simulink model "fxpdemo_diff"  (Simulink 5.0)
settings: Solver=ode5  SolverMode=SingleTasking  StartTime=0.0  StopTime=10  FixedStep=SampleTime/5  RelTol=1e-3  AbsTol=1e-6
PreLoadFcn:
  | preload_diff
values from neighbouring files (symbols this model uses):
  PoleZ = 0.85    [preload_diff.m]    (also in preload_lead_lag.m = exp( SampleTime * PoleS     ))
  SampleTime = 0.05    [preload_diff.m]    (also in preload_integrate.m; preload_lead_lag.m; preload_state_space.m = 0.01)
libraries: fixpt_lib_4 x7, simulink x1, fixpt_lib_3p1 x1
settings Model: RequirementInfo=9  CovMetricSettings=d  MinMaxOverflowLogging=MinMaxAndOverflow  Creator=andyb  LastModifiedBy=andyb  ExtModeTrigMode=oneshot  ExtModeArmWhenConnect=off  ExtModeAutoUpdateStatusClock=off  LimitDataPoints=off  IntegerOverflowMsg=none  ParameterDowncastMsg=warning  ParameterOverflowMsg=warning  ParameterPrecisionLossMsg=none  BooleanDataType=off  RTWOptions="-aEnforceIntegerDowncast=1 -aExtMode=0 -aExtModeTesting=0 -aFoldNonRolledExpr=1 -aForceParamTrailComments=0 -aGenRTModel=1 -aGenerateComments=1 -aGenerateReport=0 -aIgnoreCustomStorageClasses=1 -aIncHierarchyInIds=0 -aInlineInvariantSignals=0 -aLocalBlockOutputs=1 -aLogVarNameModifier=\"rt_\" -aRTWVerbose=1 -aRollThreshold=5 -aShowEliminatedStatements=1"

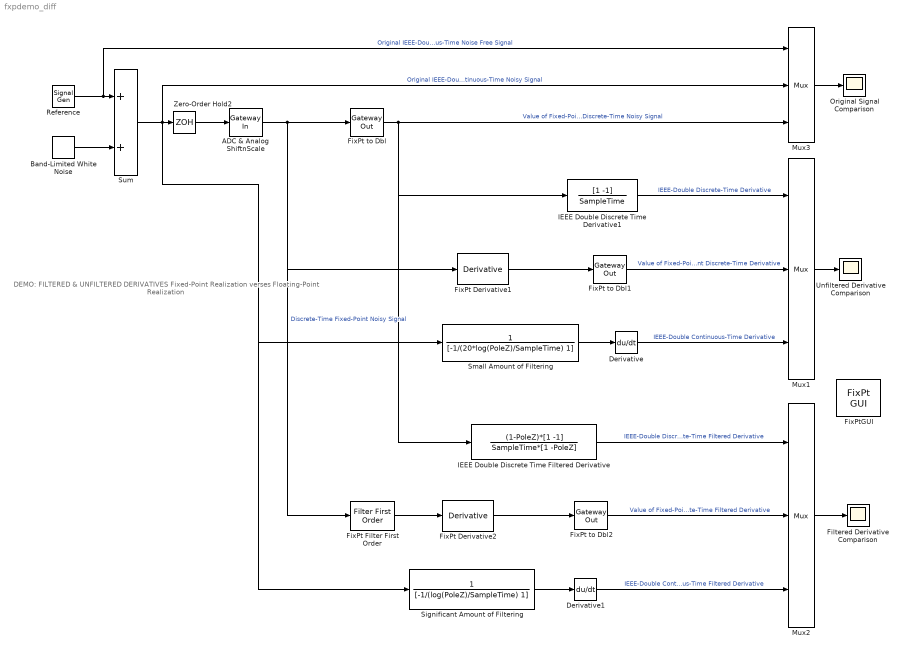
== system fxpdemo_diff ==
  note: DEMO:
      |
      | FILTERED &
      | UNFILTERED
      | DERIVATIVES
      |
      | Fixed-Point Realization
      | verses
      | Floating-Point Realization
  ADC & Analog ShiftnScale : fixpt_lib_4/Data Type/Gateway In  InRealWorld=Real World Value  OutputDataTypeScalingMode=Specify via dialog  OutDataType=sfix(16)  OutScaling=2^-9  RndMeth=Nearest  DoSatur=on
      settings: LockScale=on
  Band-Limited White Noise : simulink/Sources/Band-Limited White Noise  Cov=[0.0000005]  Ts=SampleTime/5  seed=[23341]
  Derivative : Derivative
  Derivative1 : Derivative
  Filtered Derivative Comparison : Scope
      settings: TickLabels=on  YMin=-3  YMax=3  SaveName=FiltDerivCompare
  FixPt Derivative1 : fixpt_lib_4/Calculus/Derivative  gainval=1.0  ICPrevScaledInput=0.0  OutDataType=sfix(16)  OutScaling=2^-10  DoSatur=off
  FixPt Derivative2 : fixpt_lib_4/Calculus/Derivative  gainval=1.0  ICPrevScaledInput=0.0  OutDataType=sfix(16)  OutScaling=2^-10  DoSatur=off
  FixPt Filter First Order : fixpt_lib_4/Filters/Filter First Order  PoleZ=PoleZ  ICPrevOutput=0.0  DoSatur=off
  FixPt to Dbl : fixpt_lib_4/Data Type/Gateway Out  OutRealWorld=Real World Value  OutBuiltInType=double  DoSatur=off
  FixPt to Dbl1 : fixpt_lib_4/Data Type/Gateway Out  OutRealWorld=Real World Value  OutBuiltInType=double  DoSatur=off
  FixPt to Dbl2 : fixpt_lib_4/Data Type/Gateway Out  OutRealWorld=Real World Value  OutBuiltInType=double  DoSatur=off
  FixPtGUI : fixpt_lib_3p1/FixPt GUI
  IEEE Double Discrete Time Derivative1 : DiscreteFilter  Numerator=[1 -1]  Denominator=SampleTime  SampleTime=SampleTime
  IEEE Double Discrete Time Filtered Derivative : DiscreteFilter  Numerator=(1-PoleZ)*[1 -1]  Denominator=SampleTime*[1 -PoleZ]  SampleTime=SampleTime
  Mux1 : Mux  Inputs=3
  Mux2 : Mux  Inputs=3
  Mux3 : Mux  Inputs=3
  Original Signal Comparison : Scope
      settings: TickLabels=on  YMin=-4  YMax=4  SaveName=OrigSignalCompare
  Reference : SignalGenerator  Amplitude=3  Frequency=0.1*1
  Significant Amount of Filtering : TransferFcn  Denominator=[-1/(log(PoleZ)/SampleTime) 1]
  Small Amount of Filtering : TransferFcn  Denominator=[-1/(20*log(PoleZ)/SampleTime) 1]
  Sum : Sum  Inputs=2  SaturateOnIntegerOverflow=on  InputSameDT=on
  Unfiltered Derivative Comparison : Scope
      settings: TickLabels=on  TimeRange=10  YMin=-3  YMax=3  SaveName=UnfiltDerivCompare
  Zero-Order Hold2 : ZeroOrderHold  SampleTime=SampleTime
  wires:
  Sum/1 -> Zero-Order Hold2/1, Significant Amount of Filtering/1, Mux3/2, Small Amount of Filtering/1  "Original IEEE-Double Continuous-Time Noisy Signal"
  Zero-Order Hold2/1 -> ADC & Analog ShiftnScale/1
  ADC & Analog ShiftnScale/1 -> FixPt to Dbl/1, FixPt Derivative1/1, FixPt Filter First Order/1  "Discrete-Time Fixed-Point Noisy Signal"
  FixPt to Dbl/1 -> Mux3/3, IEEE Double Discrete Time Derivative1/1, IEEE Double Discrete Time Filtered Derivative/1  "Value of Fixed-Point Discrete-Time Noisy Signal"
  FixPt Derivative1/1 -> FixPt to Dbl1/1
  FixPt to Dbl1/1 -> Mux1/2  "Value of Fixed-Point Discrete-Time Derivative"
  IEEE Double Discrete Time Derivative1/1 -> Mux1/1  "IEEE-Double Discrete-Time Derivative"
  Derivative/1 -> Mux1/3  "IEEE-Double Continuous-Time Derivative"
  Mux1/1 -> Unfiltered Derivative Comparison/1
  FixPt Filter First Order/1 -> FixPt Derivative2/1
  FixPt to Dbl2/1 -> Mux2/2  "Value of Fixed-Point Discrete-Time Filtered Derivative"
  IEEE Double Discrete Time Filtered Derivative/1 -> Mux2/1  "IEEE-Double Discrete-Time Filtered Derivative"
  Derivative1/1 -> Mux2/3  "IEEE-Double Continuous-Time Filtered Derivative"
  Significant Amount of Filtering/1 -> Derivative1/1
  Mux2/1 -> Filtered Derivative Comparison/1
  Mux3/1 -> Original Signal Comparison/1
  Small Amount of Filtering/1 -> Derivative/1
  Reference/1 -> Sum/1, Mux3/1  "Original IEEE-Double Continuous-Time Noise Free Signal"
  Band-Limited White Noise/1 -> Sum/2
  FixPt Derivative2/1 -> FixPt to Dbl2/1
